simulink model "derivador_puro_teste"  (R2017b)
settings: Solver=ode45  StartTime=0.0  StopTime=10  RelTol=1e-3
settings Model: Creator=fernandopassold  LastModifiedBy=fernandopassold

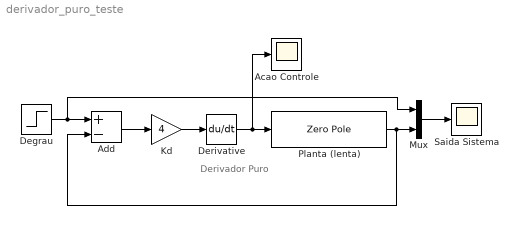
== system derivador_puro_teste ==
  note: Derivador
      | Puro
  Acao Controle : Scope
  Add : Sum  Inputs=+-
  Degrau : Step  SampleTime=0
  Derivative : Derivative
  Kd : Gain  Gain=4
  Mux : Mux  Inputs=2
  Planta (lenta) : ZeroPole  Zeros=[ ]  Poles=[-0.25]  Gain=1/4
  Saida Sistema : Scope
  wires:
  Derivative/1 -> Acao Controle/1, Planta (lenta)/1
  Degrau/1 -> Mux/1, Add/1
  Mux/1 -> Saida Sistema/1
  Planta (lenta)/1 -> Add/2, Mux/2
  Add/1 -> Kd/1
  Kd/1 -> Derivative/1
